simulink model "HW02_96101838_4_1"  (R2017a)
settings: Solver=VariableStepAuto  StartTime=-5.0  StopTime=15  RelTol=1e-3
settings Model: Creator=Micronet  LastModifiedBy=Micronet

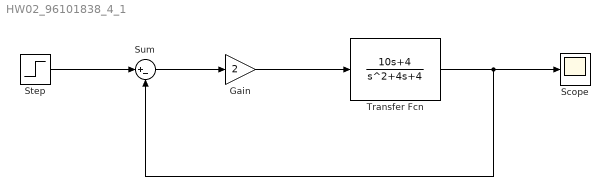
== system HW02_96101838_4_1 ==
  Gain : Gain  Gain=2
  Scope : Scope
  Step : Step  Time=0  SampleTime=0
  Sum : Sum  Inputs=|+-
  Transfer Fcn : TransferFcn  Numerator=[10 4]  Denominator=[1 4 4]
  wires:
  Gain/1 -> Transfer Fcn/1
  Transfer Fcn/1 -> Sum/2, Scope/1
  Step/1 -> Sum/1
  Sum/1 -> Gain/1
